simulink model "lunchline_ex8"  (R2016a)
settings: Solver=VariableStepAuto  StartTime=0.0  StopTime=90  RelTol=1e-3
undefined symbols (not defined in the file): m, n
libraries: simulink x1
settings Model: Creator=ningd  LastModifiedBy=ningd

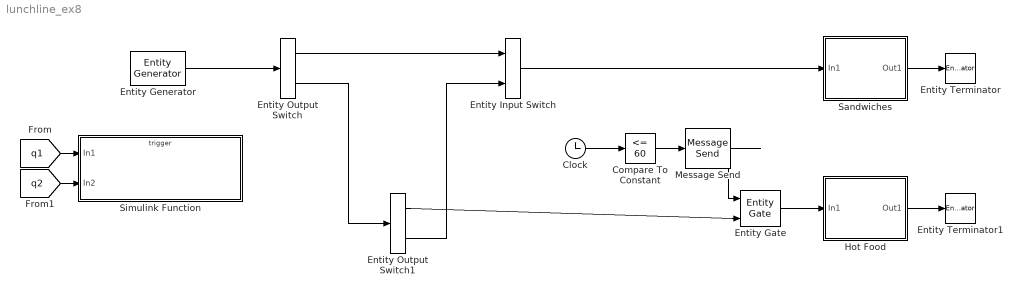
== system lunchline_ex8 ==
  Clock : Clock
  Compare To Constant : simulink/Logic and Bit Operations/Compare To Constant  relop=<=  const=60  OutDataTypeStr=boolean
  Entity Input Switch : EntityInputSwitch  InputPortMessageModes=m,m  OutputPortMessageModes=m
  Entity Output Switch : EntityOutputSwitch  InputPortMessageModes=m  OutputPortMessageModes=m,m  SwitchingCriterion=From attribute  SwitchAttributeName=Lunch
  Entity Output Switch1 : EntityOutputSwitch  InputPortMessageModes=m  OutputPortMessageModes=m,m  SwitchAttributeName=Attribute1
  Entity Gate : EntityGate  InputPortMessageModes=m,m  OutputPortMessageModes=m
  Entity Generator : EntityGenerator  OutputPortMessageModes=m  TimeSource=MATLAB action  IntergenerationTimeAction=dt = exprnd(0.5);  GenerateEntityAtSimulationStart=off  GenerateAction=|  AttributeName=ServiceTime|Lunch  AttributeInitialValue=1|1  EntityType=Structured  EntityTypeName=Customer
      | % Define a service time from a normal distribution 
      | % with mean 1.7 and std deviation 0.2
      | entity.ServiceTime = 1.7 + 0.2*randn;
      | 
      | % Define Lunch attribute using a Simulink Function 
      | % that calculates the shortest lunch line queue.
      | entity.Lunch = calcShortestQueue();
  Entity Terminator : EntityTerminator  InputPortMessageModes=m
  Entity Terminator1 : EntityTerminator  InputPortMessageModes=m
  Hot Food : Subsystem
  Message Send : MessageSend  OutputPortMessageModes=m
      settings: InputPortMap=u1
  Sandwiches : Subsystem
  Simulink Function : Subsystem  TreatAsAtomicUnit=on
  wires:
  Entity Generator/1 -> Entity Output Switch/1
  Sandwiches/1(Out1) -> Entity Terminator/1
  Hot Food/1(Out1) -> Entity Terminator1/1
  [q1] -> Simulink Function/1(In1)
  [q2] -> Simulink Function/2(In2)
  Entity Output Switch/2 -> Entity Output Switch1/1
  Clock/1 -> Compare To Constant/1
  Compare To Constant/1 -> Message Send/1
  Message Send/1 -> Entity Gate/1
  Entity Gate/1 -> Hot Food/1(In1)
  Entity Output Switch1/1 -> Entity Gate/2
  Entity Input Switch/1 -> Sandwiches/1(In1)
  Entity Output Switch/1 -> Entity Input Switch/1
  Entity Output Switch1/2 -> Entity Input Switch/2

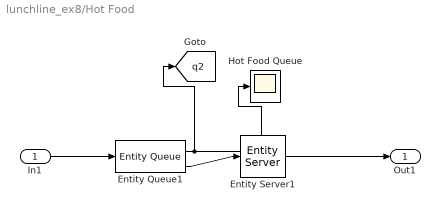
== system lunchline_ex8/Hot Food ==
  In1 : Inport
  Entity Queue1 : EntityQueue  InputPortMessageModes=m  OutputPortMessageModes=n,m  NumberEntitiesInBlock=on
      settings: OutputPortMap=o1,o5
  Entity Server1 : EntityServer  InputPortMessageModes=m  OutputPortMessageModes=m  Capacity=2  ServiceTimeSource=Attribute
  Hot Food Queue : Scope
  Out1 : Outport
  tag scope: q2=global
  wires:
  Entity Queue1/2 -> Entity Server1/1
  Entity Server1/1 -> Out1/1
  Entity Queue1/1 -> [q2], Hot Food Queue/1
  In1/1 -> Entity Queue1/1

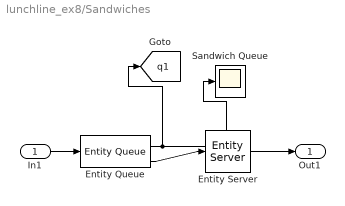
== system lunchline_ex8/Sandwiches ==
  In1 : Inport
  Entity Queue : EntityQueue  InputPortMessageModes=m  OutputPortMessageModes=n,m  NumberEntitiesInBlock=on
      settings: OutputPortMap=o1,o5
  Entity Server : EntityServer  InputPortMessageModes=m  OutputPortMessageModes=m  Capacity=2  ServiceTimeSource=Attribute
  Sandwich Queue : Scope
  Out1 : Outport
  tag scope: q1=global
  wires:
  Entity Queue/2 -> Entity Server/1
  Entity Server/1 -> Out1/1
  Entity Queue/1 -> [q1], Sandwich Queue/1
  In1/1 -> Entity Queue/1

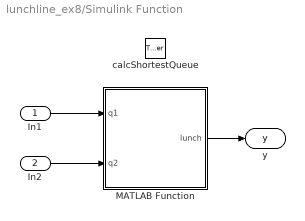
== system lunchline_ex8/Simulink Function ==
  In1 : Inport
  In2 : Inport  Port=2
  calcShortestQueue : TriggerPort  TriggerType=function-call  IsSimulinkFunction=on  FunctionName=calcShortestQueue  VariantControl=Variant
  MATLAB Function : MATLAB Function  TreatAsAtomicUnit=on
  y : ArgOut  DisableCoverage=on  ArgumentName=y
  wires:
  MATLAB Function/1(lunch) -> y/1
  In1/1 -> MATLAB Function/1(q1)
  In2/1 -> MATLAB Function/2(q2)

== matlab function lunchline_ex8/Simulink Function/MATLAB Function ==
  data: q1 input; lunch output; q2 input
function lunch = calcShortest(q1,q2)
%#codegen

if q1 < q2
    lunch = 1;              % Queue 1 is shortest
elseif q1 > q2
    lunch = 2;              % Queue 2 is shortest
else
    lunch = randi([1 2]);   % Queues are equal
end
